simulink model "Quad_Nonlinear_Roll"  (R2020a)
settings: Solver=ode4  StartTime=0.0  StopTime=10  FixedStep=0.01  RelTol=1e-3
InitFcn:
  | LQIR_Solver;
undefined symbols (not defined in the file or in its folder): Aa, g, h_cg, J_xx, K, m1, m_tot, miu_k, r_x
libraries: simulink x1, eeGeneralControl x1
settings Model: Creator=Ali  LastModifiedBy=Ali

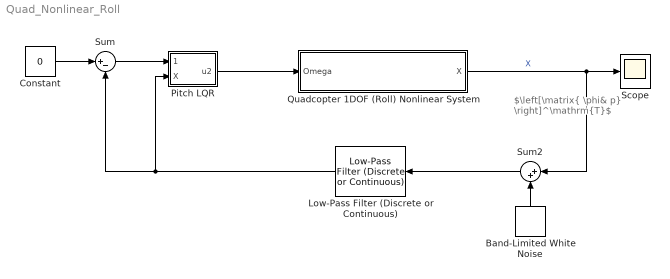
== system Quad_Nonlinear_Roll ==
  note: $\left[\matrix{ \phi& p} \right]^\mathrm{T}$
  Band-Limited White Noise : simulink/Sources/Band-Limited White Noise  Cov=[0.0001]  Ts=0.02  seed=[23341]
  Constant : Constant  Value=0
  Low-Pass Filter (Discrete or Continuous) : eeGeneralControl/Low-Pass Filter (Discrete or Continuous)  K=1  T=0.05  B=inf  A=-inf  init_option=Inherited from block input  x0=0  Ts=0
  Pitch LQR : Subsystem
  Quadcopter 1DOF (Roll) Nonlinear System : Subsystem  TreatAsAtomicUnit=on
      mask Display: image('Seesaw.png'); % Use "Edit Image" on toolstrip to change.
  Scope : Scope
  Sum : Sum  Inputs=|+-
  Sum2 : Sum  Inputs=|++
  wires:
  Band-Limited White Noise/1 -> Sum2/2
  Low-Pass Filter (Discrete or Continuous)/1 -> Pitch LQR/2(X), Sum/2
  Pitch LQR/1(u2) -> Quadcopter 1DOF (Roll) Nonlinear System/1(Omega)
  Quadcopter 1DOF (Roll) Nonlinear System/1(X) -> Sum2/1, Scope/1  "X"
  Constant/1 -> Sum/1
  Sum2/1 -> Low-Pass Filter (Discrete or Continuous)/1
  Sum/1 -> Pitch LQR/1(Error)

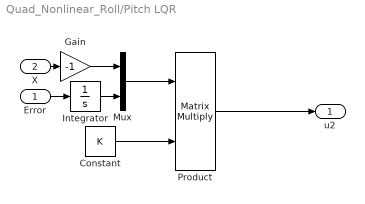
== system Quad_Nonlinear_Roll/Pitch LQR ==
  Error : Inport
  X : Inport  Port=2
  Constant : Constant  Value=K
  Gain : Gain  Gain=-1
  Integrator : Integrator
  Mux : Mux  Inputs=2
  Product : Product  Multiplication=Matrix(*)
  u2 : Outport
  wires:
  Product/1 -> u2/1
  X/1 -> Gain/1
  Error/1 -> Integrator/1
  Mux/1 -> Product/1
  Constant/1 -> Product/2
  Integrator/1 -> Mux/2
  Gain/1 -> Mux/1

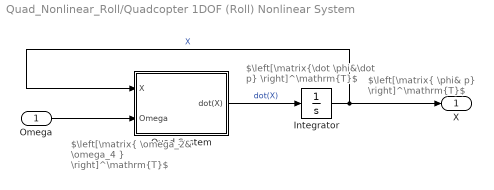
== system Quad_Nonlinear_Roll/Quadcopter 1DOF (Roll) Nonlinear System ==
  note: $\left[\matrix{ \phi& p} \right]^\mathrm{T}$
  note: $\left[\matrix{ \omega_2& \omega_4 } \right]^\mathrm{T}$
  note: $\left[\matrix{\dot \phi&\dot p} \right]^\mathrm{T}$
  Omega : Inport
  Integrator : Integrator  InitialCondition=[0.6, 1]
  Quad System : Subsystem
  X : Outport
  wires:
  Integrator/1 -> Quad System/1(X), X/1  "X"
  Quad System/1(dot(X)) -> Integrator/1  "dot(X)"
  Omega/1 -> Quad System/2(Omega)

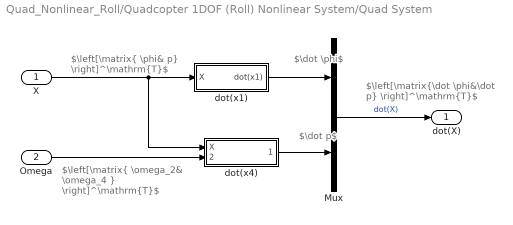
== system Quad_Nonlinear_Roll/Quadcopter 1DOF (Roll) Nonlinear System/Quad System ==
  note: $\dot \phi$
  note: $\left[\matrix{ \omega_2& \omega_4 } \right]^\mathrm{T}$
  note: $\left[\matrix{ \phi& p} \right]^\mathrm{T}$
  note: $\left[\matrix{\dot \phi&\dot p} \right]^\mathrm{T}$
  note: $\dot p$
  X : Inport
  Omega : Inport  Port=2
  Mux : Mux  Inputs=2
  dot(x1) : Subsystem
  dot(x4) : Subsystem
  dot(X) : Outport
  wires:
  Mux/1 -> dot(X)/1  "dot(X)"
  X/1 -> dot(x4)/1(X), dot(x1)/1(X)
  Omega/1 -> dot(x4)/2(Omega)
  dot(x1)/1(dot(x1)) -> Mux/1
  dot(x4)/1(dot(x4)) -> Mux/2

== system Quad_Nonlinear_Roll/Quadcopter 1DOF (Roll) Nonlinear System/Quad System/dot(x1) ==
  X : Inport
  Subsystem1 : Subsystem
  dot(x1) : Outport
  wires:
  X/1 -> Subsystem1/1(X)  "X"
  Subsystem1/1(x4) -> dot(x1)/1

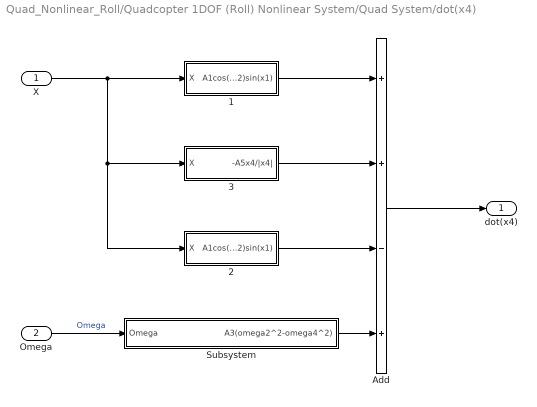
== system Quad_Nonlinear_Roll/Quadcopter 1DOF (Roll) Nonlinear System/Quad System/dot(x4) ==
  X : Inport
  Omega : Inport  Port=2
  1 : Subsystem
  2 : Subsystem
  3 : Subsystem
  Add : Sum  Inputs=++-+
  Subsystem : Subsystem
  dot(x4) : Outport
  wires:
  Omega/1 -> Subsystem/1(Omega)  "Omega"
  Add/1 -> dot(x4)/1
  1/1(A1cos(x2)sin(x1)) -> Add/1
  3/1("-A5x4/|x4| ") -> Add/2
  X/1 -> 2/1(X), 3/1(X), 1/1(X)
  Subsystem/1(A3(omega2^2-omega4^2)) -> Add/4
  2/1(A1cos(x2)sin(x1)) -> Add/3

== system Quad_Nonlinear_Roll/Quadcopter 1DOF (Roll) Nonlinear System/Quad System/dot(x1)/Subsystem1 ==
  X : Inport
  Selector : Selector  InputPortWidth=2  IndexOptions=Index vector (dialog)  Indices=[2]  OutputSizes=1
  x4 : Outport
  wires:
  Selector/1 -> x4/1
  X/1 -> Selector/1

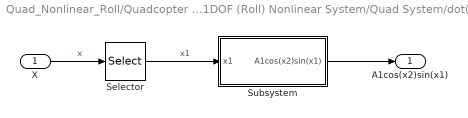
== system Quad_Nonlinear_Roll/Quadcopter 1DOF (Roll) Nonlinear System/Quad System/dot(x4)/1 ==
  X : Inport
  Selector : Selector  InputPortWidth=2  IndexOptions=Index vector (dialog)  Indices=[1]  OutputSizes=1
  Subsystem : Subsystem
  A1cos(x2)sin(x1) : Outport
  wires:
  Selector/1 -> Subsystem/1(x1)  "x1"
  Subsystem/1(A1cos(x2)sin(x1)) -> A1cos(x2)sin(x1)/1
  X/1 -> Selector/1  "x"

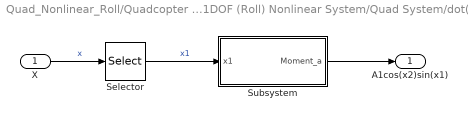
== system Quad_Nonlinear_Roll/Quadcopter 1DOF (Roll) Nonlinear System/Quad System/dot(x4)/2 ==
  X : Inport
  Selector : Selector  InputPortWidth=2  IndexOptions=Index vector (dialog)  Indices=[1]  OutputSizes=1
  Subsystem : Subsystem
  A1cos(x2)sin(x1) : Outport
  wires:
  Selector/1 -> Subsystem/1(x1)  "x1"
  Subsystem/1(Moment_a) -> A1cos(x2)sin(x1)/1
  X/1 -> Selector/1  "x"

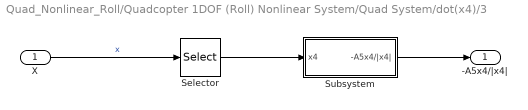
== system Quad_Nonlinear_Roll/Quadcopter 1DOF (Roll) Nonlinear System/Quad System/dot(x4)/3 ==
  X : Inport
  Selector : Selector  InputPortWidth=2  IndexOptions=Index vector (dialog)  Indices=[2]  OutputSizes=1
  Subsystem : Subsystem
  "-A5x4/|x4| " : Outport
  wires:
  Subsystem/1("-A5x4/|x4| ") -> "-A5x4/|x4| "/1
  X/1 -> Selector/1  "x"
  Selector/1 -> Subsystem/1(x4)

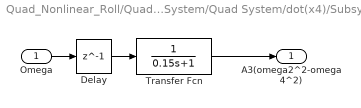
== system Quad_Nonlinear_Roll/Quadcopter 1DOF (Roll) Nonlinear System/Quad System/dot(x4)/Subsystem ==
  Omega : Inport
  Delay : Delay  DelayLength=1
  Transfer Fcn : TransferFcn  Denominator=[0.15 1]
  A3(omega2^2-omega4^2) : Outport
  wires:
  Omega/1 -> Delay/1
  Delay/1 -> Transfer Fcn/1
  Transfer Fcn/1 -> A3(omega2^2-omega4^2)/1

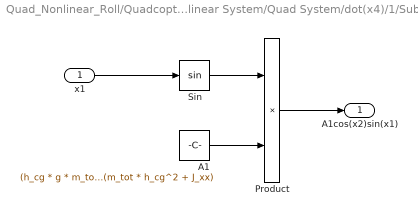
== system Quad_Nonlinear_Roll/Quadcopter 1DOF (Roll) Nonlinear System/Quad System/dot(x4)/1/Subsystem ==
  x1 : Inport
  A1 : Constant  Value=(h_cg * g * m_tot) / (m_tot * h_cg^2 + J_xx)
  Product : Product
  Sin : Trigonometry
  A1cos(x2)sin(x1) : Outport
  wires:
  Sin/1 -> Product/1
  Product/1 -> A1cos(x2)sin(x1)/1
  x1/1 -> Sin/1
  A1/1 -> Product/2

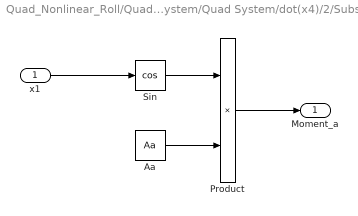
== system Quad_Nonlinear_Roll/Quadcopter 1DOF (Roll) Nonlinear System/Quad System/dot(x4)/2/Subsystem ==
  x1 : Inport
  Aa : Constant  Value=Aa
  Product : Product
  Sin : Trigonometry  Operator=cos
  Moment_a : Outport
  wires:
  Sin/1 -> Product/1
  Product/1 -> Moment_a/1
  x1/1 -> Sin/1
  Aa/1 -> Product/2

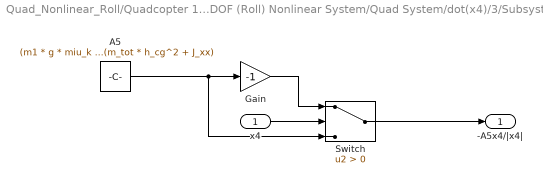
== system Quad_Nonlinear_Roll/Quadcopter 1DOF (Roll) Nonlinear System/Quad System/dot(x4)/3/Subsystem ==
  x4 : Inport
  A5 : Constant  Value=(m1 * g * miu_k * r_x) / (m_tot * h_cg^2 + J_xx)
  Gain : Gain  Gain=-1
  Switch : Switch  Criteria=u2 > Threshold
  "-A5x4/|x4| " : Outport
  wires:
  Switch/1 -> "-A5x4/|x4| "/1
  A5/1 -> Switch/3, Gain/1
  x4/1 -> Switch/2
  Gain/1 -> Switch/1
